simulink model "subsistema_termico"  (R2024b)
settings: Solver=VariableStepAuto  StartTime=0.0  StopTime=10.0  RelTol=1e-3
values from neighbouring files (symbols this model uses):
  alpha_cu = 3.9 *10^-3    (= 0.0039)    [parametros.m]
  C_ts = 0.818    [parametros.m]
  R_s_40 = 1.02    [parametros.m]
  R_ts_amb = 146.7    [parametros.m]
  Temp_s_ref = 20    [parametros.m]
settings Model: Creator=nsorr  LastModifiedBy=nsorr

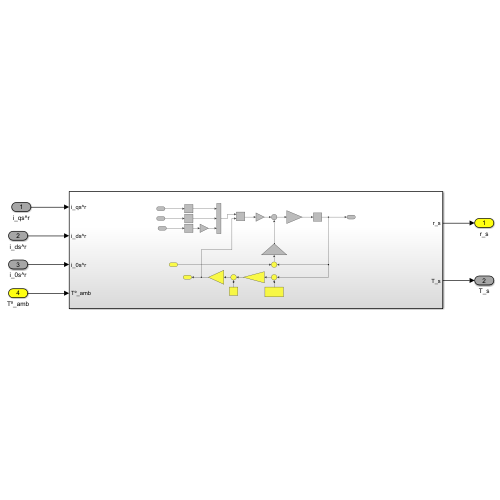
[thumbnail: Simulink's stored preview of the top-level diagram]
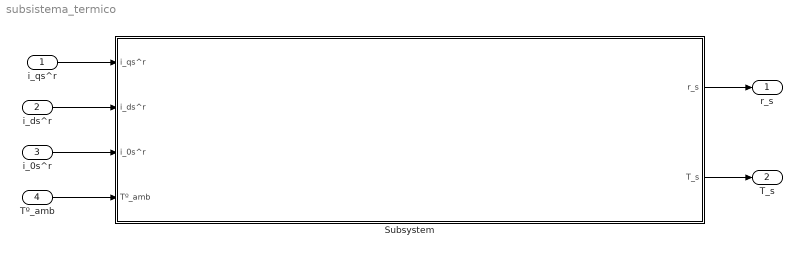
== system subsistema_termico ==
  i_qs^r : Inport
  i_ds^r : Inport  Port=2
  i_0s^r : Inport  Port=3
  Tº_amb : Inport  Port=4
  Subsystem : Subsystem
  r_s : Outport
  T_s : Outport  Port=2
  wires:
  i_qs^r/1 -> Subsystem/1(i_qs^r)
  i_ds^r/1 -> Subsystem/2(i_ds^r)
  i_0s^r/1 -> Subsystem/3(i_0s^r)
  Tº_amb/1 -> Subsystem/4(Tº_amb)
  Subsystem/1(r_s) -> r_s/1
  Subsystem/2(T_s) -> T_s/1

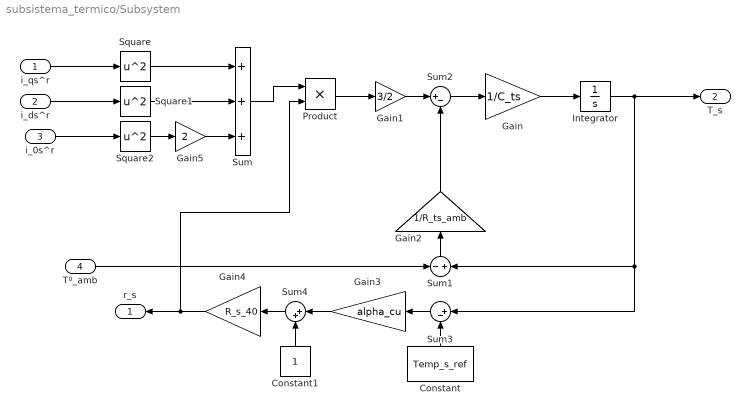
== system subsistema_termico/Subsystem ==
  i_qs^r : Inport
  i_ds^r : Inport  Port=2
  i_0s^r : Inport  Port=3
  Tº_amb : Inport  Port=4
  Constant : Constant  Value=Temp_s_ref
  Constant1 : Constant
  Gain : Gain  Gain=1/C_ts
  Gain1 : Gain  Gain=3/2
  Gain2 : Gain  Gain=1/R_ts_amb
  Gain3 : Gain  Gain=alpha_cu
  Gain4 : Gain  Gain=R_s_40
  Gain5 : Gain  Gain=2
  Integrator : Integrator  InitialCondition=40
  Product : Product
  Square : Math  Operator=square
  Square1 : Math  Operator=square
  Square2 : Math  Operator=square
  Sum : Sum  Inputs=+++
  Sum1 : Sum  Inputs=-|+
  Sum2 : Sum  Inputs=|+-
  Sum3 : Sum  Inputs=|+-
  Sum4 : Sum  Inputs=|++
  r_s : Outport
  T_s : Outport  Port=2
  wires:
  Gain4/1 -> r_s/1, Product/2
  Gain/1 -> Integrator/1
  Square/1 -> Sum/1
  i_0s^r/1 -> Square2/1
  Gain1/1 -> Sum2/1
  Sum/1 -> Product/1
  Gain3/1 -> Sum4/1
  Gain5/1 -> Sum/3
  Sum4/1 -> Gain4/1
  Gain2/1 -> Sum2/2
  Square1/1 -> Sum/2
  Constant1/1 -> Sum4/2
  Tº_amb/1 -> Sum1/1
  i_ds^r/1 -> Square1/1
  i_qs^r/1 -> Square/1
  Constant/1 -> Sum3/2
  Sum1/1 -> Gain2/1
  Sum3/1 -> Gain3/1
  Product/1 -> Gain1/1
  Integrator/1 -> T_s/1, Sum3/1, Sum1/2
  Sum2/1 -> Gain/1
  Square2/1 -> Gain5/1
